simulink model "p9_Sim_Block_Diagram"  (R2017b)
settings: Solver=ode14x  StartTime=0.0  StopTime=3  FixedStep=.001  RelTol=1e-3
settings Model: Creator=Harrison  LastModifiedBy=Harrison
settings DataIOCC: SaveFormat=Array

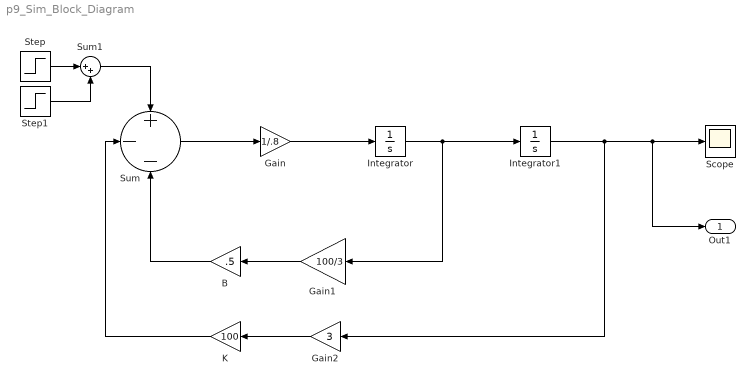
== system p9_Sim_Block_Diagram ==
  B : Gain  Gain=.5
  Gain : Gain  Gain=1/.8
  Gain1 : Gain  Gain=100/3
  Gain2 : Gain  Gain=3
  Integrator : Integrator
  Integrator1 : Integrator
  K : Gain  Gain=100
  Scope : Scope
  Step : Step  Time=0  After=10  SampleTime=0
  Step1 : Step  Time=.1  After=-10  SampleTime=0
  Sum : Sum  Inputs=+--
  Sum1 : Sum  Inputs=|++
  Out1 : Outport
  wires:
  Step/1 -> Sum1/1
  Step1/1 -> Sum1/2
  Sum1/1 -> Sum/1
  Sum/1 -> Gain/1
  Gain/1 -> Integrator/1
  Integrator/1 -> Gain1/1, Integrator1/1
  Integrator1/1 -> Gain2/1, Out1/1, Scope/1
  Gain1/1 -> B/1
  B/1 -> Sum/3
  Gain2/1 -> K/1
  K/1 -> Sum/2
